simulink model "LinearBlock"  (R2019b)
settings: Solver=VariableStepAuto  StartTime=0.0  StopTime=20.0  RelTol=1e-3
libraries: eeLuenbergerObserver x2
settings Model: Creator=marko  LastModifiedBy=marko

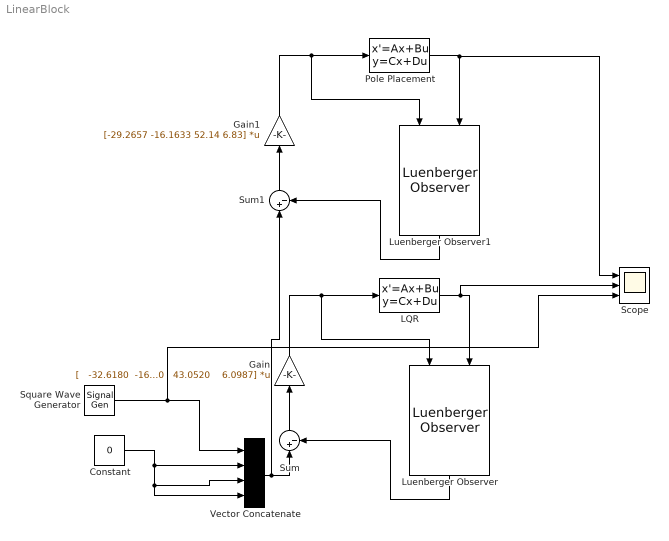
== system LinearBlock ==
  Constant : Constant  Value=0
  Gain : Gain  Gain="[   -32.6180  -16.0550   43.0520    6.0987]"  Multiplication=Matrix(K*u)
  Gain1 : Gain  Gain=[-29.2657 -16.1633 52.14 6.83]  Multiplication=Matrix(K*u)
  LQR : StateSpace  A=[0 1 0 0; 0 -1 -9.8 0; 0 0 0 1; -0.98/(0.33) 0 0 -0.1/(0.33)]  B=[0; 0; 0; 3]  C=[1 0 0 0]  D=0  InitialCondition=[0.1;0;0;0]
  Luenberger Observer : eeLuenbergerObserver/Luenberger Observer  StateSpaceType=Continuous-time  Ad=1  Bd=1  Cd=1  Dd=1  A=[0 1 0 0; 0 -1 -9.8 0; 0 0 0 1; -0.98/(0.33) 0 0 -0.1/(0.33)]  B=[0; 0; 0; 3]  C=[1 0 0 0]  D=0  ObserverDesign=Desired eigenvalues  Ld=1  DesiredEigenvalues=[-40, -50, -60, -70]  x0=[0.1; 0; 0; 0]  Tsd=0.01  Ts=0.01
      settings: SourceProductName=Simscape Electrical  SourceProductBaseCode=PS
  Luenberger Observer1 : eeLuenbergerObserver/Luenberger Observer  StateSpaceType=Continuous-time  Ad=1  Bd=1  Cd=1  Dd=1  A=[0 1 0 0; 0 -1 -9.8 0; 0 0 0 1; -0.98/(0.33) 0 0 -0.1/(0.33)]  B=[0; 0; 0; 3]  C=[1 0 0 0]  D=0  ObserverDesign=Desired eigenvalues  Ld=1  DesiredEigenvalues=[-40, -50, -60, -70]  x0=[0.1; 0; 0; 0]  Tsd=0.01  Ts=0.01
      settings: SourceProductName=Simscape Electrical  SourceProductBaseCode=PS
  Pole Placement : StateSpace  A=[0 1 0 0; 0 -1 -9.8 0; 0 0 0 1; -0.98/(0.33) 0 0 -0.1/(0.33)]  B=[0; 0; 0; 3]  C=[1 0 0 0]  D=0  InitialCondition=[0.1;0;0;0]
  Scope : Scope  NumInputPorts=3
  Square Wave Generator : SignalGenerator  WaveForm=square  Amplitude=0.1  Frequency=0.8  Units=rad/sec
  Sum : Sum  Inputs=|+-
  Sum1 : Sum  Inputs=|+-
  Vector Concatenate : Concatenate  NumInputs=4
  wires:
  LQR/1 -> Scope/2, Luenberger Observer/2
  Gain/1 -> Luenberger Observer/1, LQR/1
  Luenberger Observer/1 -> Sum/2
  Vector Concatenate/1 -> Sum/1, Sum1/1
  Sum/1 -> Gain/1
  Square Wave Generator/1 -> Scope/3, Vector Concatenate/1
  Constant/1 -> Vector Concatenate/2, Vector Concatenate/4, Vector Concatenate/3
  Sum1/1 -> Gain1/1
  Luenberger Observer1/1 -> Sum1/2
  Pole Placement/1 -> Scope/1, Luenberger Observer1/2
  Gain1/1 -> Luenberger Observer1/1, Pole Placement/1
